simulink model "untitled"  (R2024b)
settings: Solver=VariableStepAuto  StartTime=0.0  StopTime=10.0  MaxStep=1e-4  RelTol=1e-3
values from neighbouring files (symbols this model uses):
  A = [0 -(1-D_ss)/L ... (first row only)    [prelim.m]
  B = [VO_ss/L ... (first row only)    [prelim.m]
undefined symbols (not defined in the file or in its folder): K_ex
settings Model: Creator=Αναστασία Λίβα  LastModifiedBy=Αναστασία Λίβα

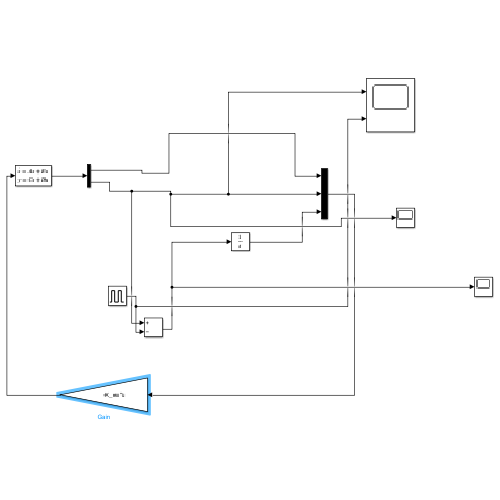
[thumbnail: Simulink's stored preview of the top-level diagram]
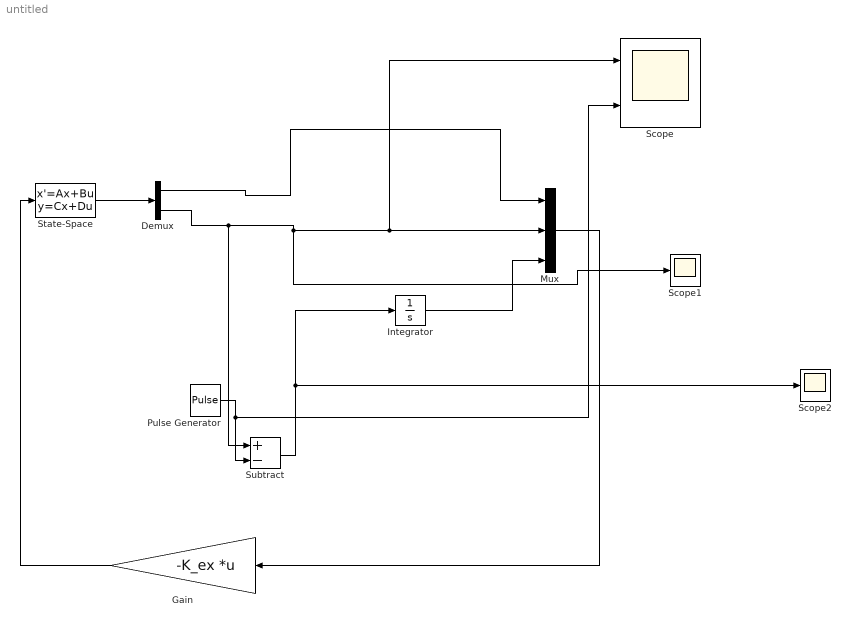
== system untitled ==
  Demux : Demux  Outputs=2
  Gain : Gain  Gain=-K_ex  Multiplication=Matrix(K*u)
  Integrator : Integrator
  Mux : Mux  Inputs=3
  Pulse Generator : DiscretePulseGenerator  PulseType=Time based  Period=3  PulseWidth=30
  Scope : Scope  NumInputPorts=2
  Scope1 : Scope
  Scope2 : Scope
  State-Space : StateSpace  A=A  B=B  C=eye(2)  D=[0;0]  InitialCondition="[2  0]"
  Subtract : Sum  Inputs=+-
  wires:
  State-Space/1 -> Demux/1
  Demux/2 -> Scope1/1, Scope/1, Mux/2, Subtract/1
  Mux/1 -> Gain/1
  Gain/1 -> State-Space/1
  Demux/1 -> Mux/1
  Integrator/1 -> Mux/3
  Subtract/1 -> Integrator/1, Scope2/1
  Pulse Generator/1 -> Scope/2, Subtract/2
